simulink model "Q3_e"  (R2022a)
settings: Solver=FixedStepDiscrete  StartTime=0.0  StopTime=10.0  FixedStep=0.1  RelTol=1e-3  EnableMultiTasking=on
settings Model: FPTShortcutValueString='{{},{''BaselineRun'',1,1,1,''BaselineRun'','''',{},''M'','''',''''},{''BaselineRun_2'',1,1,1,''BaselineRun_2'','''',{},''M'','''',''''}}'  ExtModeTrigDuration=2  Creator=Erfan  LastModifiedBy=Erfan
settings SolverCC: AlgebraicLoopSolver=TrustRegion  AutoInsertRateTranBlk=on
settings DataIOCC: LimitDataPoints=on
settings OptimizationCC: EnhancedBackFolding=on  PassReuseOutputArgsAs=Individual arguments  ZeroExternalMemoryAtStartup=off  ZeroInternalMemoryAtStartup=off  MaxStackSize=64  OptimizeBlockOrder=speed  DifferentSizesBufferReuse=on  OptimizationCustomize=off  EfficientTunableParamExpr=on
settings DebuggingCC: SignalRangeChecking=warning  ParameterTunabilityLossMsg=error  UnconnectedInputMsg=warning  UnconnectedOutputMsg=warning  UnconnectedLineMsg=warning  AllowSymbolicDim=off  SFUnexpectedBacktrackingDiag=warning  SFNoUnconditionalDefaultTransitionDiag=warning  SFExecutionAtInitializationDiag=none  ArithmeticOperatorsInVariantConditions=warning
settings HardwareCC: ProdBitPerInt=16  ProdBitPerPointer=16  ProdBitPerSizeT=16  ProdBitPerPtrDiffT=16  ProdLargestAtomicFloat=None  ProdWordSize=8  ProdHWDeviceType=Atmel->AVR
settings SFSimCC: SimUseLocalCustomCode=off  MATLABDynamicMemAlloc=off  CustomCodeUndefinedFunction=UseInterfaceOnly
settings RTWCC: SystemTargetFile=ert.tlc  HardwareBoard=Arduino Mega 2560  TemplateMakefile=ert_default_tmf  RTWUseLocalCustomCode=off  Toolchain=Arduino AVR  DLArmComputeVersion=19.05
settings CodeAppCC: ForceParamTrailComments=on  IgnoreCustomStorageClasses=off  OperatorAnnotations=on  SimulinkDataObjDesc=on  SFDataObjDesc=on  InsertBlockDesc=on
settings ERTTargetCC: TargetLangStandard=C99 (ISO)  SupportContinuousTime=on  SupportVariableSizeSignals=on  ExtModeTransport=3  ExtModeStaticAlloc=on  ExtModeStaticAllocSize=2048  ExtModeMexFile=ext_xcp  ExtModeIntrfLevel=Level2 - Open
settings ConfigComp: CovMetricSettings=dw  CovSaveCumulativeToWorkspaceVar=on  CovSaveSingleToWorkspaceVar=on  CovExternalEMLEnable=off  CovSFcnEnable=off

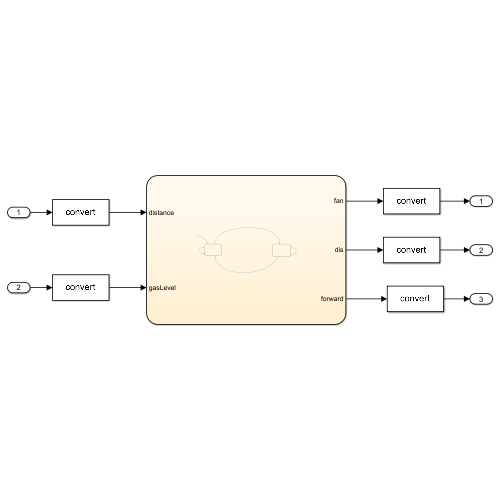
[thumbnail: Simulink's stored preview of the top-level diagram]
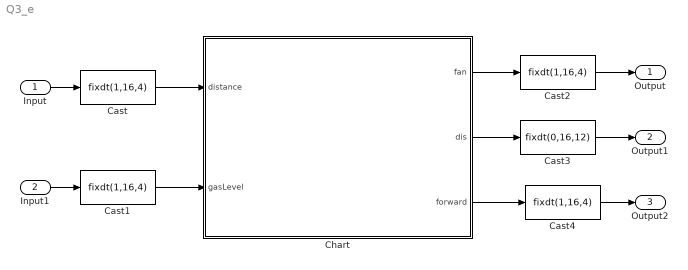
== system Q3_e ==
  Input : Inport  OutDataTypeStr=fixdt(1,16,4)
  Input1 : Inport  Port=2  OutDataTypeStr=fixdt(1,16,4)
  Cast{,1..2,4} (4 alike) : DataTypeConversion  OutDataTypeStr=fixdt(1,16,4)  SaturateOnIntegerOverflow=off  RndMeth=Floor
  Cast3 : DataTypeConversion  OutDataTypeStr=fixdt(0,16,12)  SaturateOnIntegerOverflow=off  RndMeth=Floor
  Chart : Stateflow chart  TreatAsAtomicUnit=on
  Output : Outport
  Output1 : Outport  Port=2
  Output2 : Outport  Port=3
  wires:
  Chart/1(fan) -> Cast2/1
  Input/1 -> Cast/1
  Input1/1 -> Cast1/1
  Chart/3(forward) -> Cast4/1
  Chart/2(dis) -> Cast3/1
  Cast/1 -> Chart/1(distance)
  Cast1/1 -> Chart/2(gasLevel)
  Cast2/1 -> Output/1
  Cast3/1 -> Output1/1
  Cast4/1 -> Output2/1

== stateflow chart Q3_e/Chart ==
  state Forward_Moving
    during:
    fan = 1;
    forward = 1;
  state Backward_Moving
    during:
    fan = 0;
    forward = -1;
  Forward_Moving -> Backward_Moving [order 1] : [gasLevel > 100 || distance < 100  ]
  (default) -> Forward_Moving
  Backward_Moving -> Backward_Moving [order 2] : [gasLevel >= 100 && distance <= 100 ]{dis = dis -1;}
  Forward_Moving -> Forward_Moving [order 2] : [gasLevel <= 100 &&  distance >= 100 ]{dis = dis + 1;}
  Backward_Moving -> Forward_Moving [order 1] : [gasLevel < 100 || distance > 100 ]
  data: distance input; fan output; gasLevel input; dis output =10; forward output
